simulink model "lqr"  (R2024a)
settings: Solver=VariableStepAuto  StartTime=0.0  StopTime=10.0  RelTol=10e-7
values from neighbouring files (symbols this model uses):
  A = [4, -2, 0, 6; -2, 4, -6, 0; 0, -6, 4, 2; 6, 0, 2, 4]    [main.m]
  C = [1, -1, 1, 1; 1, 3, -1, 3]    [main.m]
  L = -P * C' / R    [TAU.m]    (also in main.m = TAU.FindObserverKalman(A, C, QL, RL))
  varf = 1    [main.m]
  x0 = [1; 1; 1; 1]    [main.m]
settings Model: Creator=alexivanov  LastModifiedBy=alexivanov

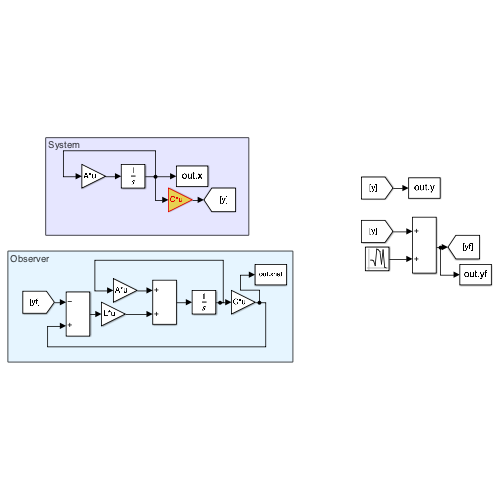
[thumbnail: Simulink's stored preview of the top-level diagram]
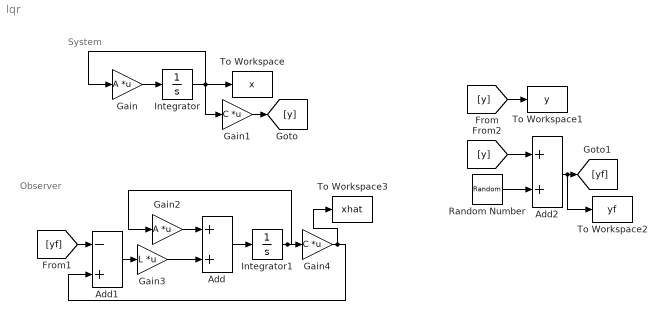
== system lqr ==
  note: Observer
  note: System
  Add : Sum
  Add1 : Sum  Inputs=-+
  Add2 : Sum
  Gain : Gain  Gain=A  Multiplication=Matrix(K*u)
  Gain1 : Gain  Gain=C  Multiplication=Matrix(K*u)
  Gain2 : Gain  Gain=A  Multiplication=Matrix(K*u)
  Gain3 : Gain  Gain=L  Multiplication=Matrix(K*u)
  Gain4 : Gain  Gain=C  Multiplication=Matrix(K*u)
  Integrator : Integrator  InitialCondition=x0
  Integrator1 : Integrator
  Random Number : RandomNumber  Variance=varf  SampleTime=0.001
  To Workspace : ToWorkspace  VariableName=x  SampleTime=-1
  To Workspace1 : ToWorkspace  VariableName=y  SampleTime=-1
  To Workspace2 : ToWorkspace  VariableName=yf  SampleTime=-1
  To Workspace3 : ToWorkspace  VariableName=xhat  SampleTime=-1
  wires:
  Gain/1 -> Integrator/1
  Integrator/1 -> Gain1/1, To Workspace/1, Gain/1
  Gain1/1 -> [y]
  [y] -> To Workspace1/1
  Gain2/1 -> Add/1
  Add/1 -> Integrator1/1
  Integrator1/1 -> Gain2/1, Gain4/1
  Gain3/1 -> Add/2
  Add1/1 -> Gain3/1
  [yf] -> Add1/1
  Gain4/1 -> To Workspace3/1, Add1/2
  [y] -> Add2/1
  Random Number/1 -> Add2/2
  Add2/1 -> To Workspace2/1, [yf]
